simulink model "Introduction_to_Simulink"  (R2015a)
settings: Solver=ode45  StartTime=0.0  StopTime=10.0  RelTol=1e-3
settings Model: Creator=aidanlaw  LastModifiedBy=aidanlaw

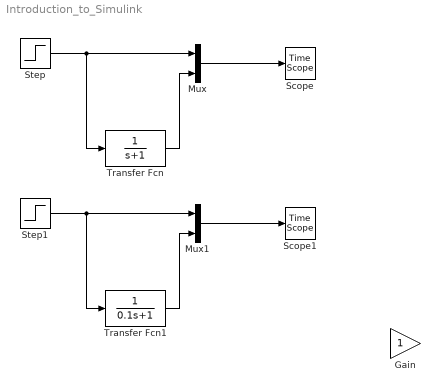
== system Introduction_to_Simulink ==
  Gain : Gain
  Mux : Mux  Inputs=2
  Mux1 : Mux  Inputs=2
  Scope : TimeScope
  Scope1 : TimeScope
  Step : Step  SampleTime=0
  Step1 : Step  SampleTime=0
  Transfer Fcn : TransferFcn  Denominator=[1 1]
  Transfer Fcn1 : TransferFcn  Denominator=[0.1 1]
  wires:
  Step/1 -> Transfer Fcn/1, Mux/1
  Transfer Fcn/1 -> Mux/2
  Mux/1 -> Scope/1
  Step1/1 -> Transfer Fcn1/1, Mux1/1
  Transfer Fcn1/1 -> Mux1/2
  Mux1/1 -> Scope1/1
